simulink model "control_model"  (R2018a)
settings: Solver=FixedStepAuto  StartTime=0.0  StopTime=50  FixedStep=Te
values from neighbouring files (symbols this model uses):
  f = 0.0001    [IM_model.m]    (also in transfer_function.m)
  J = 0.011    [IM_model.m]    (also in transfer_function.m)
  Lr = 0.0302409    [IM_model.m]    (also in transfer_function.m)
  Ls = 0.0302409    [IM_model.m]    (also in transfer_function.m)
  p = 1    [IM_model.m]    (also in transfer_function.m)
  Rr = 10.3654    [IM_model.m]    (also in transfer_function.m)
  Rs = 11    [IM_model.m]    (also in transfer_function.m)
  Te = 10^-4    (= 0.0001)    [IM_model.m]    (also in data_aquisition11.m = 0.001)
libraries: powerlib x16, pePwmGenerator x3, simulink x1
settings Model: Creator=ali  LastModifiedBy=ali

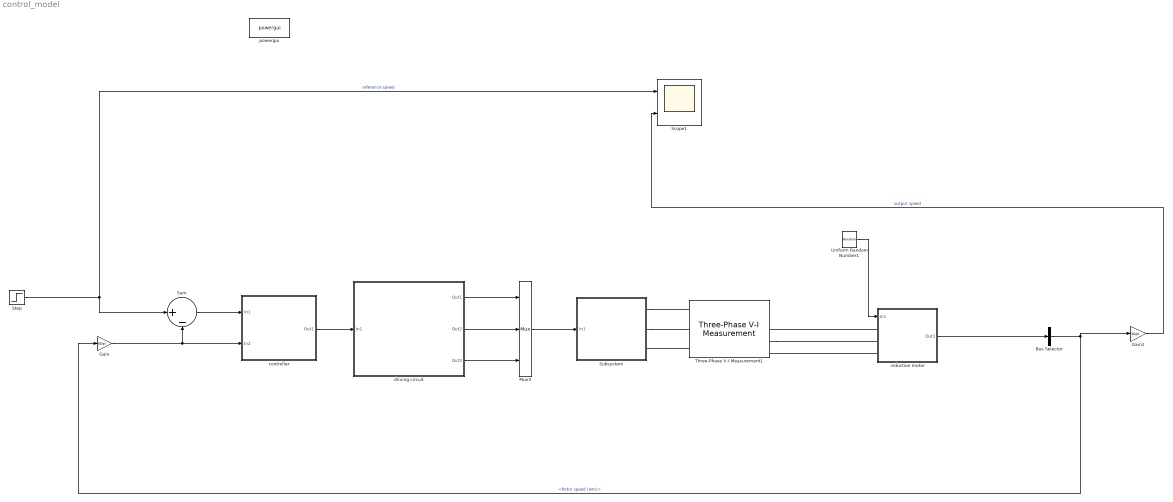
== system control_model ==
  Bus Selector : BusSelector  OutputSignals=Mechanical.Rotor speed (wm)
  Gain : Gain  Gain=30/pi
  Gain1 : Gain  Gain=30/pi
  Mux3 : Mux  Inputs=3
  Scope1 : Scope  NumInputPorts=2
  Step : Step  Time=0  After=1500  SampleTime=0
  Subsystem : Subsystem
  Sum : Sum  Inputs=|+-
  Three-Phase V-I Measurement1 : powerlib/Measurements/Three-Phase V-I Measurement  VoltageMeasurement=phase-to-phase  SetLabelV=off  LabelV=Vabc  Vpu=off  VpuLL=off  CurrentMeasurement=yes  SetLabelI=off  LabelI=Iabc  Ipu=off  Pbase=100e6  Vbase=500e3  OutputType=Complex  PhasorSimulation=off  PSBequivalent=0
  Uniform Random Number1 : UniformRandomNumber  Minimum=1500  Maximum=2500  SampleTime=10
  controller : Subsystem
  driving circuit : Subsystem
  induction motor : Subsystem
  powergui : powerlib/powergui  Priority=1  SimulationMode=Discrete  SampleTime=Te  frequency=60  Iterations=50  frequencyindice=0  Pbase=100e6  ErrMax=1e-4  UnitsV=kV  UnitsW=MW  buscounter=0  FunctionMessages=off  echomessages=off  EnableUseOfTLC=off  CurrentSourceSwitches=off  DisableSnubberDevices=off  DisableRonSwitches=off  DisableVfSwitches=off  DisplayEquations=off  SolverType=Tustin/Backward Euler (TBE)  Interpol=off  ExternalGateDelay=off  methode=off  Ts=100  x0status=blocks  SPID=off  SwTol=0  HookPort=off  RestoreLinks=warning  ResistiveCurrentMeasurement=off  Frange=[0:2:500]  Ylog=off  Xlog=on  ShowGrid=off  save=off  variable=ZData  structure=0  ZoomFFT=off  StartTime=0.0  cycles=1  DisplayStyle=1  fundamental=60  FreqAxis=off  MaxFrequency=1000  frequencyindicesteady=1  RmsSteady=1  display=off
  wires:
  Bus Selector/1 -> Gain1/1, Gain/1  "<Rotor speed (wm)>"
  Gain/1 -> controller/2(In2), Sum/2
  Step/1 -> Sum/1, Scope1/1  "reference speed"
  Gain1/1 -> Scope1/2  "output speed"
  induction motor/1(Out1) -> Bus Selector/1
  Sum/1 -> controller/1(In1)
  Uniform Random Number1/1 -> induction motor/1(In1)
  Mux3/1 -> Subsystem/1(In1)
  controller/1(Out1) -> driving circuit/1(In1)
  driving circuit/1(Out1) -> Mux3/1
  driving circuit/2(Out2) -> Mux3/2
  driving circuit/3(Out3) -> Mux3/3
  connections:
  induction motor/LConn1 -- Three-Phase V-I Measurement1/RConn1
  Three-Phase V-I Measurement1/RConn2 -- induction motor/LConn2
  induction motor/LConn3 -- Three-Phase V-I Measurement1/RConn3
  Subsystem/RConn1 -- Three-Phase V-I Measurement1/LConn1
  Subsystem/RConn2 -- Three-Phase V-I Measurement1/LConn2
  Three-Phase V-I Measurement1/LConn3 -- Subsystem/RConn3

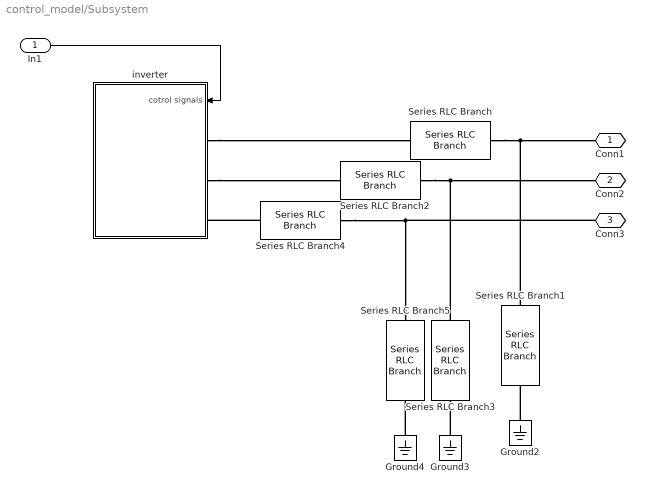
== system control_model/Subsystem ==
  In1 : Inport
  Ground2 : powerlib/Elements/Ground  LConnTagsString=a
  Ground3 : powerlib/Elements/Ground  LConnTagsString=a
  Ground4 : powerlib/Elements/Ground  LConnTagsString=a
  Series RLC Branch : powerlib/Elements/Series RLC Branch  LConnTagsString=__new0  RConnTagsString=__new0  BranchType=L  Resistance=1  Inductance=10e-3  SetiL0=off  InitialCurrent=0  Capacitance=1e-6  Setx0=off  InitialVoltage=0  Measurements=None
  Series RLC Branch1 : powerlib/Elements/Series RLC Branch  LConnTagsString=__new0  RConnTagsString=__new0  BranchType=C  Resistance=1  Inductance=1e-3  SetiL0=off  InitialCurrent=0  Capacitance=440e-6  Setx0=off  InitialVoltage=0  Measurements=None
  Series RLC Branch2 : powerlib/Elements/Series RLC Branch  LConnTagsString=__new0  RConnTagsString=__new0  BranchType=L  Resistance=1  Inductance=10e-3  SetiL0=off  InitialCurrent=0  Capacitance=1e-6  Setx0=off  InitialVoltage=0  Measurements=None
  Series RLC Branch3 : powerlib/Elements/Series RLC Branch  LConnTagsString=__new0  RConnTagsString=__new0  BranchType=C  Resistance=1  Inductance=1e-3  SetiL0=off  InitialCurrent=0  Capacitance=440e-6  Setx0=off  InitialVoltage=0  Measurements=None
  Series RLC Branch4 : powerlib/Elements/Series RLC Branch  LConnTagsString=__new0  RConnTagsString=__new0  BranchType=L  Resistance=1  Inductance=10e-3  SetiL0=off  InitialCurrent=0  Capacitance=1e-6  Setx0=off  InitialVoltage=0  Measurements=None
  Series RLC Branch5 : powerlib/Elements/Series RLC Branch  LConnTagsString=__new0  RConnTagsString=__new0  BranchType=C  Resistance=1  Inductance=1e-3  SetiL0=off  InitialCurrent=0  Capacitance=440e-6  Setx0=off  InitialVoltage=0  Measurements=None
  inverter : Subsystem
  Conn1 : PMIOPort  Side=Right
  Conn2 : PMIOPort  Port=2  Side=Right
  Conn3 : PMIOPort  Port=3  Side=Right
  wires:
  In1/1 -> inverter/1("cotrol signals ")
  connections:
  Ground3/LConn1 -- Series RLC Branch3/RConn1
  Series RLC Branch/RConn1 -- Conn1/RConn1 -- Series RLC Branch1/LConn1
  Series RLC Branch2/RConn1 -- Conn2/RConn1 -- Series RLC Branch3/LConn1
  Ground2/LConn1 -- Series RLC Branch1/RConn1
  Ground4/LConn1 -- Series RLC Branch5/RConn1
  Series RLC Branch4/LConn1 -- inverter/LConn3
  Series RLC Branch4/RConn1 -- Conn3/RConn1 -- Series RLC Branch5/LConn1
  inverter/LConn2 -- Series RLC Branch2/LConn1
  inverter/LConn1 -- Series RLC Branch/LConn1

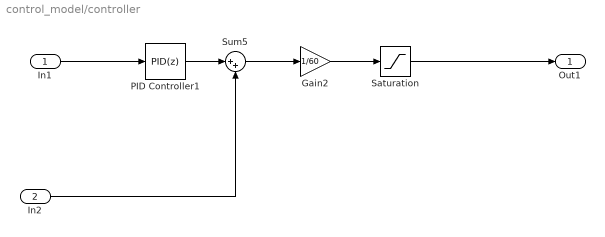
== system control_model/controller ==
  In1 : Inport
  In2 : Inport  Port=2
  Gain2 : Gain  Gain=1/60
  PID Controller1 : simulink/Continuous/PID Controller  Controller=PID  TimeDomain=Discrete-time  SampleTime=1e-4  IntegratorMethod=Forward Euler  FilterMethod=Forward Euler  Form=Parallel  UseFilter=on  ControllerParametersSource=internal  P=2.5  I=1.4  D=0  N=100  InitialConditionSource=internal  InitialConditionForIntegrator=0  InitialConditionForFilter=0  ExternalReset=none  LimitOutput=off  UpperSaturationLimit=inf  LowerSaturationLimit=-inf  LinearizeAsGain=on  AntiWindupMode=none  Kb=1  TrackingMode=off  Kt=1  PParamMin=[]  PParamMax=[]  IParamMin=[]  IParamMax=[]  DParamMin=[]  DParamMax=[]  NParamMin=[]  NParamMax=[]  KbParamMin=[]  KbParamMax=[]  KtParamMin=[]  KtParamMax=[]  POutMin=[]  POutMax=[]  IOutMin=[]  IOutMax=[]  DOutMin=[]  DOutMax=[]  NOutMin=[]  NOutMax=[]  KbOutMin=[]  KbOutMax=[]  KtOutMin=[]  KtOutMax=[]  IntegratorOutMin=[]  IntegratorOutMax=[]  FilterOutMin=[]  FilterOutMax=[]  SumOutMin=[]  SumOutMax=[]  SumI1OutMin=[]  SumI1OutMax=[]  SumI2OutMin=[]  SumI2OutMax=[]  SumI3OutMin=[]  SumI3OutMax=[]  SumDOutMin=[]  SumDOutMax=[]  SaturationOutMin=[]  SaturationOutMax=[]  IntegratorContinuousStateAttributes=''  IntegratorStateMustResolveToSignalObject=off  IntegratorRTWStateStorageClass=Auto  FilterContinuousStateAttributes=''  FilterStateMustResolveToSignalObject=off  FilterRTWStateStorageClass=Auto  DifferentiatorICPrevScaledInput=0  DifferentiatorOutMin=[]  DifferentiatorOutMax=[]  FilterDiffOutCoefMin=[]  FilterDiffOutCoefMax=[]  SumDenOutMin=[]  SumDenOutMax=[]  SumNumOutMin=[]  SumNumOutMax=[]  ReciprocalOutMin=[]  ReciprocalOutMax=[]  DivideOutMin=[]  DivideOutMax=[]  TunerSelectOption=Transfer Function Based (PID Tuner App)
  Saturation : Saturate  UpperLimit=50  LowerLimit=10
  Sum5 : Sum  Inputs=|++
  Out1 : Outport
  wires:
  PID Controller1/1 -> Sum5/1
  In2/1 -> Sum5/2
  Saturation/1 -> Out1/1
  Sum5/1 -> Gain2/1
  Gain2/1 -> Saturation/1
  In1/1 -> PID Controller1/1

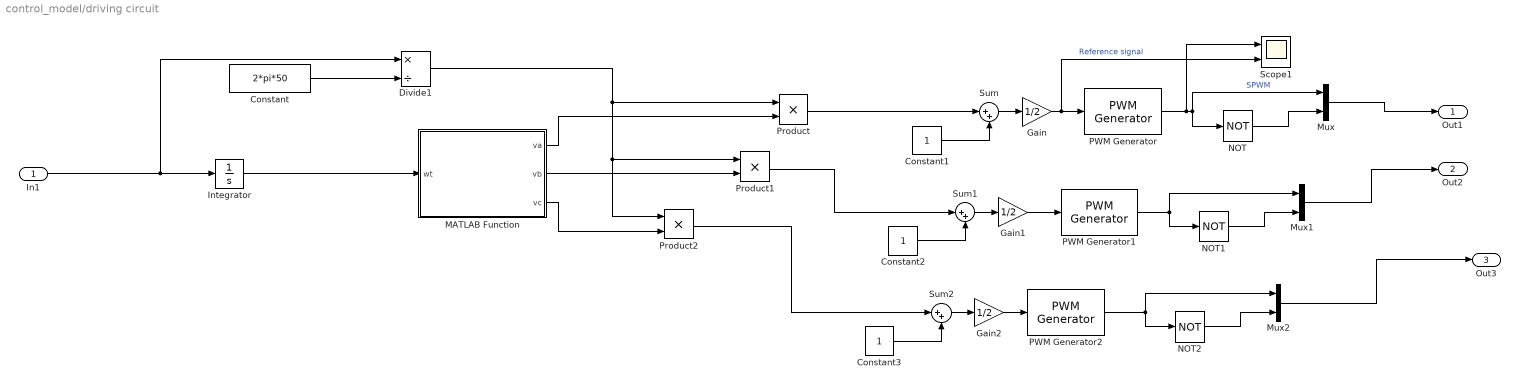
== system control_model/driving circuit ==
  In1 : Inport
  Constant : Constant  Value=2*pi*50
  Constant1 : Constant
  Constant2 : Constant
  Constant3 : Constant
  Divide1 : Product  Inputs=*/
  Gain : Gain  Gain=1/2
  Gain1 : Gain  Gain=1/2
  Gain2 : Gain  Gain=1/2
  Integrator : Integrator
  MATLAB Function : MATLAB Function  TreatAsAtomicUnit=on
  Mux : Mux  Inputs=2
  Mux1 : Mux  Inputs=2
  Mux2 : Mux  Inputs=2
  NOT : Logic  Operator=NOT  IconShape=distinctive  AllPortsSameDT=off  OutDataTypeStr=boolean
  NOT1 : Logic  Operator=NOT  IconShape=distinctive  AllPortsSameDT=off  OutDataTypeStr=boolean
  NOT2 : Logic  Operator=NOT  IconShape=distinctive  AllPortsSameDT=off  OutDataTypeStr=boolean
  PWM Generator : pePwmGenerator/PWM Generator  CarrCount=Up  Tper=10*Te  Ts=Te
  PWM Generator1 : pePwmGenerator/PWM Generator  CarrCount=Up  Tper=10*Te  Ts=Te
  PWM Generator2 : pePwmGenerator/PWM Generator  CarrCount=Up  Tper=10*Te  Ts=Te
  Product : Product
  Product1 : Product
  Product2 : Product
  Scope1 : Scope  NumInputPorts=2
  Sum : Sum  Inputs=|++
  Sum1 : Sum  Inputs=|++
  Sum2 : Sum  Inputs=|++
  Out1 : Outport
  Out2 : Outport  Port=2
  Out3 : Outport  Port=3
  wires:
  MATLAB Function/1(va) -> Product/2
  Product1/1 -> Sum1/1
  Gain2/1 -> PWM Generator2/1
  Gain1/1 -> PWM Generator1/1
  Constant3/1 -> Sum2/2
  PWM Generator2/1 -> Mux2/1, NOT2/1
  Mux1/1 -> Out2/1
  MATLAB Function/3(vc) -> Product2/2
  Constant2/1 -> Sum1/2
  PWM Generator1/1 -> Mux1/1, NOT1/1
  Sum2/1 -> Gain2/1
  PWM Generator/1 -> Scope1/1, Mux/1, NOT/1  "SPWM"
  NOT/1 -> Mux/2
  Mux/1 -> Out1/1
  Mux2/1 -> Out3/1
  NOT1/1 -> Mux1/2
  Constant/1 -> Divide1/2
  Gain/1 -> PWM Generator/1, Scope1/2  "Reference signal"
  Sum1/1 -> Gain1/1
  Integrator/1 -> MATLAB Function/1(wt)
  In1/1 -> Integrator/1, Divide1/1
  Constant1/1 -> Sum/2
  MATLAB Function/2(vb) -> Product1/2
  Divide1/1 -> Product/1, Product2/1, Product1/1
  NOT2/1 -> Mux2/2
  Product/1 -> Sum/1
  Product2/1 -> Sum2/1
  Sum/1 -> Gain/1

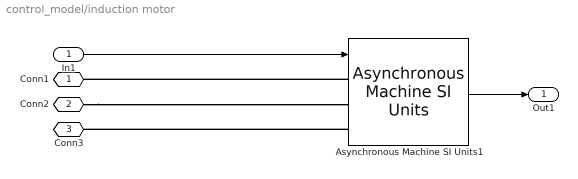
== system control_model/induction motor ==
  In1 : Inport
  Asynchronous Machine SI Units1 : powerlib/Machines/Asynchronous Machine SI Units  RotorType=Squirrel-cage  PresetModel=No  MechanicalLoad=Torque Tm  ShowDetailedParameters=on  ReferenceFrame=Rotor  Units=SI  MeasurementBus=off  NominalParameters=[630 460 50]  Stator=[Rs Ls]  Rotor=[Rr Lr]  Cage1=[0.4155 0.002066]  Cage2=[0.4168 0.0003495]  Lm=Msr  Mechanical=[J f p]  PolePairs=2  InitialConditions=[0 0 0 0 0 0 0 0]  SimulateSaturation=off  Saturation=[14.03593122, 27.81365428, 53.79336849, 72.68890987, 97.98006896, 148.6815601, 215.7428561, 302.9841135, 428.7778367 ; 230, 322, 414, 460, 506, 552, 598, 644, 690]  LoadFlowParameters=1492000  TsPowergui=0  TsBlock=1e-4  IterativeModel=Trapezoidal non iterative  IterativeDiscreteModel=Trapezoidal non iterative  Pmec=1.492e+006
  Conn1 : PMIOPort  Side=Left
  Conn2 : PMIOPort  Port=2  Side=Left
  Conn3 : PMIOPort  Port=3  Side=Left
  Out1 : Outport
  wires:
  In1/1 -> Asynchronous Machine SI Units1/1
  Asynchronous Machine SI Units1/1 -> Out1/1
  connections:
  Asynchronous Machine SI Units1/LConn1 -- Conn1/RConn1
  Conn2/RConn1 -- Asynchronous Machine SI Units1/LConn2
  Asynchronous Machine SI Units1/LConn3 -- Conn3/RConn1

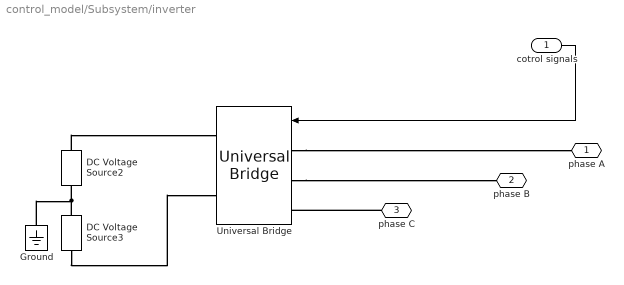
== system control_model/Subsystem/inverter ==
  "cotrol signals " : Inport
  DC Voltage Source2 : powerlib/Electrical Sources/DC Voltage Source  Amplitude=sqrt(2)*120  Measurements=None
  DC Voltage Source3 : powerlib/Electrical Sources/DC Voltage Source  Amplitude=sqrt(2)*120  Measurements=None
  Ground : powerlib/Elements/Ground  LConnTagsString=a
  Universal Bridge : powerlib/Power Electronics/Universal Bridge  Arms=3  SnubberResistance=1e5  SnubberCapacitance=inf  Device=IGBT / Diodes  Ron=1e-3  Lon=0  ForwardVoltages="[  0  0  ]"  ForwardVoltage=0  GTOparameters=[ 10e-6 , 20e-6 ]  IGBTparameters=[ 1e-6 , 2e-6 ]  Measurements=None  Measurements_2=None  converterType=Rectifier
  phase A : PMIOPort  Side=Left
  phase B : PMIOPort  Port=2  Side=Left
  phase C : PMIOPort  Port=3  Side=Left
  wires:
  "cotrol signals "/1 -> Universal Bridge/1
  connections:
  Universal Bridge/LConn1 -- phase A/RConn1
  DC Voltage Source3/RConn1 -- Ground/LConn1 -- DC Voltage Source2/LConn1
  DC Voltage Source3/LConn1 -- Universal Bridge/RConn2
  phase C/RConn1 -- Universal Bridge/LConn3
  DC Voltage Source2/RConn1 -- Universal Bridge/RConn1
  Universal Bridge/LConn2 -- phase B/RConn1

== matlab function control_model/driving circuit/MATLAB Function ==
  data: wt input; va output; vb output; vc output
function [va, vb, vc] = ThreePhaseSine(wt)

    va = sin(wt);
    vb = sin(wt - 2*pi/3);
    vc = sin(wt - 4*pi/3);
end
